simulink model "vfs_matlab"  (R2022a)
settings: Solver=FixedStepAuto  StartTime=0.0  StopTime=tend  FixedStep=0.01  RelTol=1e-3
undefined symbols (not defined in the file): Angle, Axis, center, epsilon, gd, Homogeneous, Kc, pwo_init, scale, SE3, v
libraries: simlib_vpc_basic x23, simlib_vpc_coremath x13, simlib_vpc_gp x3
settings Model: Creator=marco  LastModifiedBy=marco
settings DebuggingCC: AlgebraicLoopMsg=none  ArtificialAlgebraicLoopMsg=none  UnconnectedInputMsg=warning  UnconnectedOutputMsg=warning  UnconnectedLineMsg=warning
settings RTWCC: DLArmComputeVersion=19.05

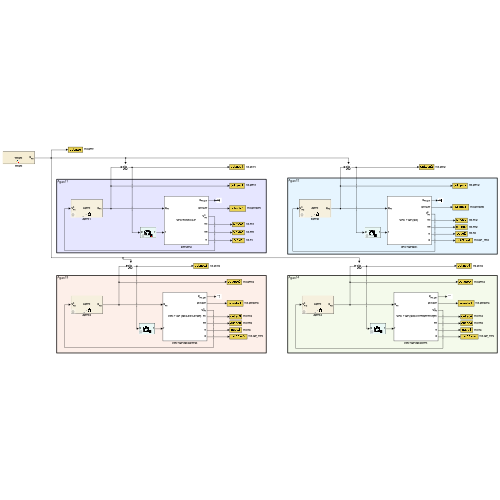
[thumbnail: Simulink's stored preview of the top-level diagram]
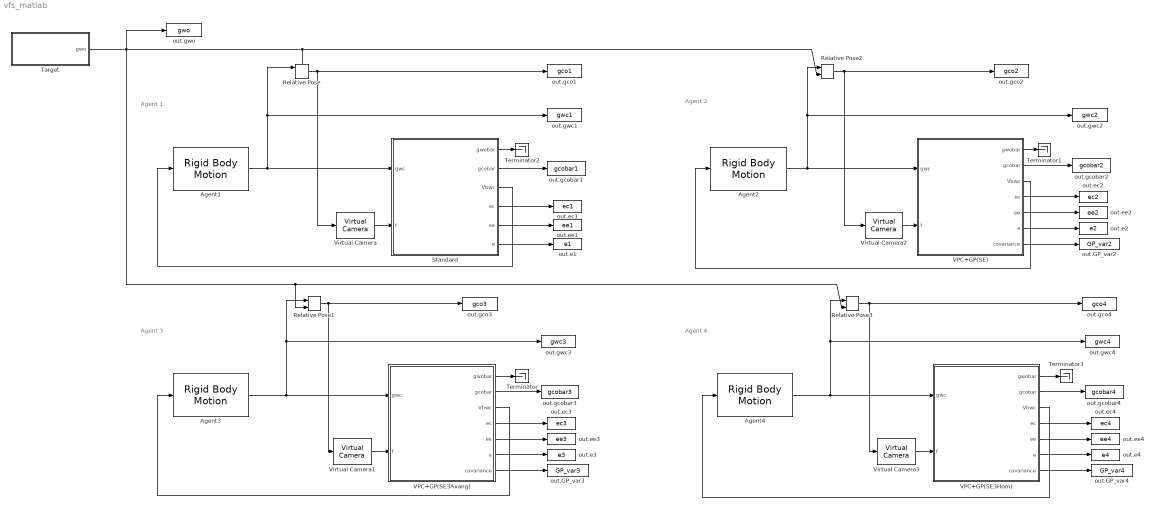
== system vfs_matlab ==
  note: Agent 3
  note: Agent 2
  note: Agent 1
  note: Agent 4
  Agent1 : simlib_vpc_basic/Rigid Body Motion  rbmtype=agent  agentnumber=1  projection=on  show_dg=off  g0=gwc_init
      settings: SourceProductName=VPC Library
  Agent2 : simlib_vpc_basic/Rigid Body Motion  rbmtype=agent  agentnumber=2  projection=on  show_dg=off  g0=gwc_init
      settings: SourceProductName=VPC Library
  Agent3 : simlib_vpc_basic/Rigid Body Motion  rbmtype=agent  agentnumber=3  projection=on  show_dg=off  g0=gwc_init
      settings: SourceProductName=VPC Library
  Agent4 : simlib_vpc_basic/Rigid Body Motion  rbmtype=agent  agentnumber=3  projection=on  show_dg=off  g0=gwc_init
      settings: SourceProductName=VPC Library
  Relative Pose{,1..3} (4 alike) : simlib_vpc_coremath/Relative Pose
      settings: SourceProductName=VPC Library
  Standard : Subsystem
      mask Display:
      | disp('VPC without GP','texmode','on')
      | 
      | % Label ports
      | port_label('input',1,'g_{wc}','texmode','on')
      | port_label('input',2,'f','texmode','on')
      | port_label('output',1,'g_{wo,bar}','texmode','on')
      | port_label('output',2,'gco,bar','texmode','on')
      | port_label('output',3,'V^b_{wc}','texmode','on')
      | port_label('output',4,'ec','texmode','on')
      | port_label('output',5,'ee','texmode','on')
      | port_label('output',6,'e','texmode','on')
  Target : Subsystem
      mask Display:
      | % Glitch in Matlab: If you define a line whose starting point and end point
      | % is equal, then the entire mask block is plotted in bold
      | plot([0,0],[0,0])
      | 
      | % Draw Box
      | plot([0,1,1,0,0],[0,0,1,1,0])
      | 
      | % Write label
      | disp('Target','texmode','on')
      | 
      | % Image
      | p=get_param(gcb,'Position');
      | size = min(p(3:4)-p(1:2));
      | blkscale = abs((p(3)-p(1)) / (p(4)-p(2)));
      | if abs((p(3)-p(1))) > abs((p(4)-p(2))) % block is horizontal
      |     scale = .5*[1/blkscale .6];
      | else % block is vertical
      |     scale = .5*[1 .6*blkscale];
      | end
      | pos = [1-scale(1) 0.1]/2;
      | image('ico_target.png',[pos scale],'off')
      | 
      | % Label ports
      | port_label('output',1,['g_{wo}'],'texmode','on')
  Terminator{,1..3} (4 alike) : Terminator
  VPC+GP(SE) : Subsystem
      mask Display:
      | disp('VPC + GP (SE)','texmode','on')
      | 
      | % Label ports
      | port_label('input',1,'g_{wc}','texmode','on')
      | port_label('input',2,'f','texmode','on')
      | port_label('output',1,'g_{wo,bar}','texmode','on')
      | port_label('output',2,'gco,bar','texmode','on')
      | port_label('output',3,'V^b_{wc}','texmode','on')
      | port_label('output',4,'ec','texmode','on')
      | port_label('output',5,'ee','texmode','on')
      | port_label('output',6,'e','texmode','on')
      | port_label('output',7,'\Sigma','texmode','on')
  VPC+GP(SE3Axang) : Subsystem
      mask Display:
      | disp('VPC + GP (SE3 Axis-Angle)','texmode','on')
      | 
      | % Label ports
      | port_label('input',1,'g_{wc}','texmode','on')
      | port_label('input',2,'f','texmode','on')
      | port_label('output',1,'g_{wo,bar}','texmode','on')
      | port_label('output',2,'gco,bar','texmode','on')
      | port_label('output',3,'V^b_{wc}','texmode','on')
      | port_label('output',4,'ec','texmode','on')
      | port_label('output',5,'ee','texmode','on')
      | port_label('output',6,'e','texmode','on')
      | port_label('output',7,'\Sigma','texmode','on')
  VPC+GP(SE3Hom) : Subsystem
      mask Display:
      | disp('VPC + GP (SE3 Homogeneous)','texmode','on')
      | 
      | % Label ports
      | port_label('input',1,'g_{wc}','texmode','on')
      | port_label('input',2,'f','texmode','on')
      | port_label('output',1,'g_{wo,bar}','texmode','on')
      | port_label('output',2,'gco,bar','texmode','on')
      | port_label('output',3,'V^b_{wc}','texmode','on')
      | port_label('output',4,'ec','texmode','on')
      | port_label('output',5,'ee','texmode','on')
      | port_label('output',6,'e','texmode','on')
      | port_label('output',7,'\Sigma','texmode','on')
  Virtual Camera{,1..3} (4 alike) : simlib_vpc_basic/Virtual Camera  camtype=Pinhole  po=fp  lambda=lambda
      settings: SourceProductName=VPC Library
  out.GP_var2 : ToWorkspace  VariableName=GP_var2  SaveFormat=Structure With Time  SampleTime=-1
  out.GP_var3 : ToWorkspace  VariableName=GP_var3  SaveFormat=Structure With Time  SampleTime=-1
  out.GP_var4 : ToWorkspace  VariableName=GP_var4  SaveFormat=Structure With Time  SampleTime=-1
  out.e1 : ToWorkspace  VariableName=e1  SaveFormat=Structure With Time  SampleTime=-1
  out.e2 : ToWorkspace  VariableName=e2  SaveFormat=Structure With Time  SampleTime=-1
  out.e3 : ToWorkspace  VariableName=e3  SaveFormat=Structure With Time  SampleTime=-1
  out.e4 : ToWorkspace  VariableName=e4  SaveFormat=Structure With Time  SampleTime=-1
  out.ec1 : ToWorkspace  VariableName=ec1  SaveFormat=Structure With Time  SampleTime=-1
  out.ec2 : ToWorkspace  VariableName=ec2  SaveFormat=Structure With Time  SampleTime=-1
  out.ec3 : ToWorkspace  VariableName=ec3  SaveFormat=Structure With Time  SampleTime=-1
  out.ec4 : ToWorkspace  VariableName=ec4  SaveFormat=Structure With Time  SampleTime=-1
  out.ee1 : ToWorkspace  VariableName=ee1  SaveFormat=Structure With Time  SampleTime=-1
  out.ee2 : ToWorkspace  VariableName=ee2  SaveFormat=Structure With Time  SampleTime=-1
  out.ee3 : ToWorkspace  VariableName=ee3  SaveFormat=Structure With Time  SampleTime=-1
  out.ee4 : ToWorkspace  VariableName=ee4  SaveFormat=Structure With Time  SampleTime=-1
  out.gco1 : ToWorkspace  VariableName=gco1  SaveFormat=Structure With Time  SampleTime=-1
  out.gco2 : ToWorkspace  VariableName=gco2  SaveFormat=Structure With Time  SampleTime=-1
  out.gco3 : ToWorkspace  VariableName=gco3  SaveFormat=Structure With Time  SampleTime=-1
  out.gco4 : ToWorkspace  VariableName=gco4  SaveFormat=Structure With Time  SampleTime=-1
  out.gcobar1 : ToWorkspace  VariableName=gcobar1  SaveFormat=Structure With Time  SampleTime=-1
  out.gcobar2 : ToWorkspace  VariableName=gcobar2  SaveFormat=Structure With Time  SampleTime=-1
  out.gcobar3 : ToWorkspace  VariableName=gcobar3  SaveFormat=Structure With Time  SampleTime=-1
  out.gcobar4 : ToWorkspace  VariableName=gcobar4  SaveFormat=Structure With Time  SampleTime=-1
  out.gwc1 : ToWorkspace  VariableName=gwc1  SaveFormat=Structure With Time  SampleTime=-1
  out.gwc2 : ToWorkspace  VariableName=gwc2  SaveFormat=Structure With Time  SampleTime=-1
  out.gwc3 : ToWorkspace  VariableName=gwc3  SaveFormat=Structure With Time  SampleTime=-1
  out.gwc4 : ToWorkspace  VariableName=gwc4  SaveFormat=Structure With Time  SampleTime=-1
  out.gwo : ToWorkspace  VariableName=gwo  SaveFormat=Structure With Time  SampleTime=-1
  wires:
  Relative Pose2/1 -> Virtual Camera2/1, out.gco2/1
  Relative Pose/1 -> Virtual Camera/1, out.gco1/1
  VPC+GP(SE)/2(gcobar) -> out.gcobar2/1
  VPC+GP(SE3Axang)/4(ec) -> out.ec3/1
  Relative Pose1/1 -> out.gco3/1, Virtual Camera1/1
  Agent3/1 -> VPC+GP(SE3Axang)/1(gwc), out.gwc3/1, Relative Pose1/1
  Virtual Camera/1 -> Standard/2(f)
  VPC+GP(SE3Axang)/2(gcobar) -> out.gcobar3/1
  Virtual Camera2/1 -> VPC+GP(SE)/2(f)
  VPC+GP(SE3Axang)/5(ee) -> out.ee3/1
  VPC+GP(SE)/4(ec) -> out.ec2/1
  VPC+GP(SE3Axang)/6(e) -> out.e3/1
  Virtual Camera1/1 -> VPC+GP(SE3Axang)/2(f)
  Agent1/1 -> Standard/1(gwc), out.gwc1/1, Relative Pose/1
  Standard/6(e) -> out.e1/1
  Target/1(gwo) -> out.gwo/1, Relative Pose2/2, Relative Pose/2, Relative Pose3/2, Relative Pose1/2
  Standard/4(ec) -> out.ec1/1
  Standard/5(ee) -> out.ee1/1
  Agent2/1 -> VPC+GP(SE)/1(gwc), out.gwc2/1, Relative Pose2/1
  Standard/2(gcobar) -> out.gcobar1/1
  VPC+GP(SE)/5(ee) -> out.ee2/1
  VPC+GP(SE)/6(e) -> out.e2/1
  Standard/3(Vbwc) -> Agent1/1
  VPC+GP(SE3Axang)/3(Vbwc) -> Agent3/1
  VPC+GP(SE)/3(Vbwc) -> Agent2/1
  VPC+GP(SE3Axang)/1(gwobar) -> Terminator/1
  VPC+GP(SE)/1(gwobar) -> Terminator1/1
  Standard/1(gwobar) -> Terminator2/1
  VPC+GP(SE)/7(covariance) -> out.GP_var2/1
  VPC+GP(SE3Axang)/7(covariance) -> out.GP_var3/1
  VPC+GP(SE3Hom)/6(e) -> out.e4/1
  VPC+GP(SE3Hom)/5(ee) -> out.ee4/1
  VPC+GP(SE3Hom)/2(gcobar) -> out.gcobar4/1
  VPC+GP(SE3Hom)/3(Vbwc) -> Agent4/1
  Virtual Camera3/1 -> VPC+GP(SE3Hom)/2(f)
  Agent4/1 -> VPC+GP(SE3Hom)/1(gwc), Relative Pose3/1, out.gwc4/1
  VPC+GP(SE3Hom)/4(ec) -> out.ec4/1
  Relative Pose3/1 -> Virtual Camera3/1, out.gco4/1
  VPC+GP(SE3Hom)/7(covariance) -> out.GP_var4/1
  VPC+GP(SE3Hom)/1(gwobar) -> Terminator3/1

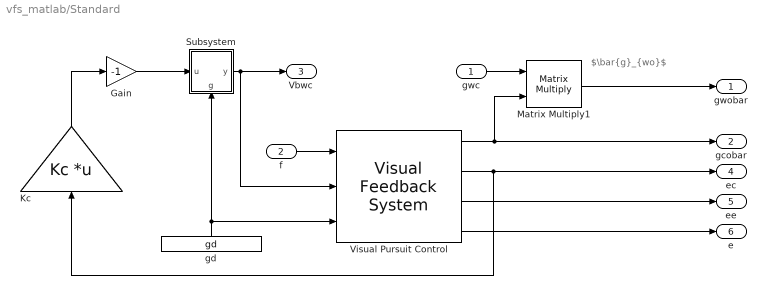
== system vfs_matlab/Standard ==
  note: $\bar{g}_{wo}$
  gwc : Inport
  f : Inport  Port=2
  Gain : Gain  Gain=-1
  Kc : Gain  Gain=Kc  Multiplication=Matrix(K*u) (u vector)
  Matrix Multiply1 : Product  Multiplication=Matrix(*)
  Subsystem : Subsystem
      settings: PortSchema="{\"entries\":[{\"content\":{\"sides\":[{\"content\":{\"connectorIds\":[\"In1\"]},\"type\":\"ConnectorPlacement.EquallySpacedRectSide\",\"uuid\":\"72e68008-5c4a-43a9-a560-64c6a31a0c08\"},{\"content\":{\"connectorIds\":[\"Out1\"],\"side\":\"RIGHT\"},\"type\":\"ConnectorPlacement.EquallySpacedRectSide\",\"uuid\":\"da07f5ff-2b2c-4c55-a2f2-34e133777503\"},{\"content\":{\"connectorIds\":[],\"side\":\"TOP\"},\"type\":\"ConnectorPlacement.EquallySpacedRectSide\",\"uuid\":\"6d174428-4364-4e89-aba7-4e9864808ab5\"},{\"content\":{\"connectorIds\":[\"In2\"],\"side\":\"BOTTOM\"},\"type\":\"ConnectorPlacement.EquallySpacedRectSide\",\"uuid\":\"f9633104-9c11-4d21-90a7-e0f886d9e92d\"},{\"content\":{\"connectorIds\":[],\"side\":\"HIDDEN\"},\"type\":\"ConnectorPlacement.EquallySpacedRectSide\",\"uuid\":\"662f08ae-9279-4a4f-85ea-81d97ead27d9\"}]},\"type\":\"ConnectorPlacement.EquallySpacedConnector\",\"uuid\":\"f3cd156c-cccd-47c6-b81c-6113f78efd58\"}],\"packageUris\":[\"http://schema.mathworks.com/mf0/Connector/R2020b\"],\"version\":\"1.0\"}"
      mask Display:
      | % Glitch in Matlab: If you define a line whose starting point and end point
      | % is equal, then the entire mask block is plotted in bold
      | plot([0,0],[0,0])
      | 
      | % Draw box
      | indent = 0.3;
      | ang=[0:0.2:pi/2, pi/2];
      | plot([0,1-indent],[0,0])
      | xp=indent*sin(ang)+1-indent;
      | yp=indent-indent*cos(ang);
      | plot(xp,yp);
      | plot([1,1,indent],[indent,1,1])
      | xp=indent-indent*sin(ang);
      | yp=1-indent+indent*cos(ang);
      | plot(xp,yp);
      | plot([0,0],[1-indent,0])
      | 
      | % Write label & ports
      | disp('-Ad_{(g_d)}','texmode','on')
      | text(0.5,0.2,'\fontsize{7}g_d','texmode','on')
  Visual Pursuit Control : simlib_vpc_basic/Visual Feedback System  gd_source=external  gd_value=[eye(4,3),ones(4,1)]  gcobar0=gco_init  Ke_source=internal  Ke=Ke  projection=on  camtype=Pinhole  fo=fp  lambda=lambda  show_Vbwo=off  show_ec=on  show_gce=off  show_ee=on  show_gee=off  show_e=on  show_nu=off  show_dgcobar=off  show_ue_aux=off
      settings: SourceProductName=VPC Library
  gd : Constant  Value=gd
  gwobar : Outport
  gcobar : Outport  Port=2
  Vbwc : Outport  Port=3
  ec : Outport  Port=4
  ee : Outport  Port=5
  e : Outport  Port=6
  wires:
  f/1 -> Visual Pursuit Control/1
  Matrix Multiply1/1 -> gwobar/1
  Subsystem/1(y) -> Vbwc/1, Visual Pursuit Control/2
  gwc/1 -> Matrix Multiply1/1
  Kc/1 -> Gain/1
  Visual Pursuit Control/4 -> e/1
  Gain/1 -> Subsystem/1(u)
  Visual Pursuit Control/2 -> ec/1, Kc/1
  Visual Pursuit Control/3 -> ee/1
  gd/1 -> Subsystem/2(g), Visual Pursuit Control/3
  Visual Pursuit Control/1 -> gcobar/1, Matrix Multiply1/2

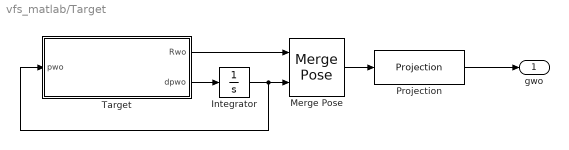
== system vfs_matlab/Target ==
  Integrator : Integrator  InitialCondition=pwo_init  ContinuousStateAttributes='pose'
  Merge Pose : simlib_vpc_coremath/Merge Pose
      settings: SourceProductName=VPC Library
  Projection : simlib_vpc_basic/Projection  projectiontype=averaging  inputtype=pose
      settings: SourceProductName=VPC Library
  Target : MATLAB Function  TreatAsAtomicUnit=on
  gwo : Outport
  wires:
  Merge Pose/1 -> Projection/1
  Projection/1 -> gwo/1
  Integrator/1 -> Target/1(pwo), Merge Pose/2
  Target/2(dpwo) -> Integrator/1
  Target/1(Rwo) -> Merge Pose/1

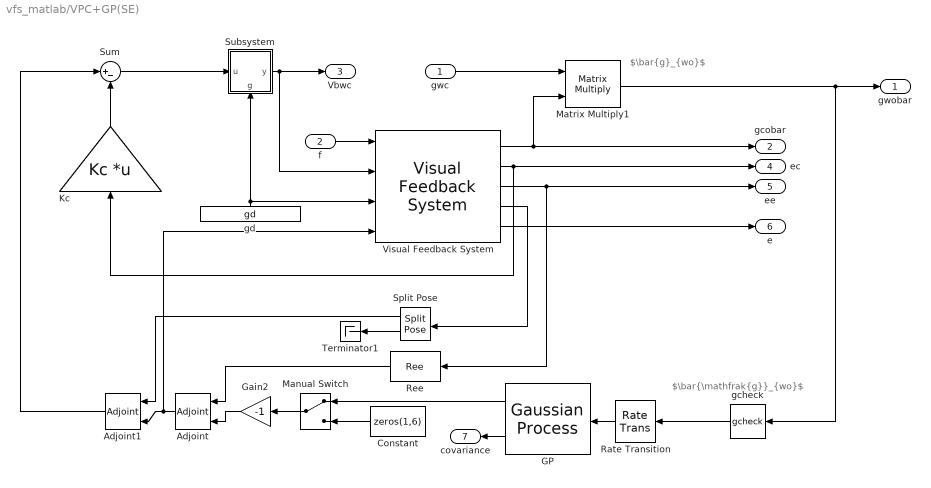
== system vfs_matlab/VPC+GP(SE) ==
  note: $\bar{g}_{wo}$
  note: $\bar{\mathfrak{g}}_{wo}$
  gwc : Inport
  f : Inport  Port=2
  Adjoint : simlib_vpc_basic/Adjoint  adjointtype=orientation
      settings: SourceProductName=VPC Library
  Adjoint1 : simlib_vpc_basic/Adjoint  adjointtype=orientation
      settings: SourceProductName=VPC Library
  Constant : Constant  Value=zeros(1,6)
  GP : simlib_vpc_gp/Gaussian Process  X=X_GP_se  Y=Y_GP_se  sn=sn_GP_se  kernel=Squared Exponential  hyp=hyp_GP_se  show_mean=on  show_variance=on  inv_fallback=off
      settings: SourceProductName=VPC Library
  Gain2 : Gain  Gain=-1
  Kc : Gain  Gain=Kc  Multiplication=Matrix(K*u) (u vector)
  Manual Switch : ManualSwitch
  Matrix Multiply1 : Product  Multiplication=Matrix(*)
  Rate Transition : RateTransition
  Ree : simlib_vpc_coremath/Ree
      settings: SourceProductName=VPC Library
  Split Pose : simlib_vpc_coremath/Split Pose  show_R=on  show_p=on
      settings: SourceProductName=VPC Library
  Subsystem : Subsystem
      settings: PortSchema="{\"entries\":[{\"content\":{\"sides\":[{\"content\":{\"connectorIds\":[\"In1\"]},\"type\":\"ConnectorPlacement.EquallySpacedRectSide\",\"uuid\":\"72e68008-5c4a-43a9-a560-64c6a31a0c08\"},{\"content\":{\"connectorIds\":[\"Out1\"],\"side\":\"RIGHT\"},\"type\":\"ConnectorPlacement.EquallySpacedRectSide\",\"uuid\":\"da07f5ff-2b2c-4c55-a2f2-34e133777503\"},{\"content\":{\"connectorIds\":[],\"side\":\"TOP\"},\"type\":\"ConnectorPlacement.EquallySpacedRectSide\",\"uuid\":\"6d174428-4364-4e89-aba7-4e9864808ab5\"},{\"content\":{\"connectorIds\":[\"In2\"],\"side\":\"BOTTOM\"},\"type\":\"ConnectorPlacement.EquallySpacedRectSide\",\"uuid\":\"f9633104-9c11-4d21-90a7-e0f886d9e92d\"},{\"content\":{\"connectorIds\":[],\"side\":\"HIDDEN\"},\"type\":\"ConnectorPlacement.EquallySpacedRectSide\",\"uuid\":\"662f08ae-9279-4a4f-85ea-81d97ead27d9\"}]},\"type\":\"ConnectorPlacement.EquallySpacedConnector\",\"uuid\":\"f3cd156c-cccd-47c6-b81c-6113f78efd58\"}],\"packageUris\":[\"http://schema.mathworks.com/mf0/Connector/R2020b\"],\"version\":\"1.0\"}"
      mask Display:
      | % Glitch in Matlab: If you define a line whose starting point and end point
      | % is equal, then the entire mask block is plotted in bold
      | plot([0,0],[0,0])
      | 
      | % Draw box
      | indent = 0.3;
      | ang=[0:0.2:pi/2, pi/2];
      | plot([0,1-indent],[0,0])
      | xp=indent*sin(ang)+1-indent;
      | yp=indent-indent*cos(ang);
      | plot(xp,yp);
      | plot([1,1,indent],[indent,1,1])
      | xp=indent-indent*sin(ang);
      | yp=1-indent+indent*cos(ang);
      | plot(xp,yp);
      | plot([0,0],[1-indent,0])
      | 
      | % Write label & ports
      | disp('-Ad_{(g_d)}','texmode','on')
      | text(0.5,0.2,'\fontsize{7}g_d','texmode','on')
  Sum : Sum  Inputs=|+-
  Terminator1 : Terminator
  Visual Feedback System : simlib_vpc_basic/Visual Feedback System  gd_source=external  gd_value=[eye(4,3),ones(4,1)]  gcobar0=gco_init  Ke_source=internal  Ke=Ke  projection=on  camtype=Pinhole  fo=fp  lambda=lambda  show_Vbwo=off  show_ec=on  show_gce=on  show_ee=on  show_gee=off  show_e=on  show_nu=off  show_dgcobar=off  show_ue_aux=on
      settings: SourceProductName=VPC Library
  gcheck : simlib_vpc_coremath/gcheck
      settings: SourceProductName=VPC Library
  gd : Constant  Value=gd
  gwobar : Outport
  gcobar : Outport  Port=2
  Vbwc : Outport  Port=3
  ec : Outport  Port=4
  ee : Outport  Port=5
  e : Outport  Port=6
  covariance : Outport  Port=7
  wires:
  f/1 -> Visual Feedback System/1
  Matrix Multiply1/1 -> gcheck/1, gwobar/1
  Subsystem/1(y) -> Vbwc/1, Visual Feedback System/2
  gwc/1 -> Matrix Multiply1/1
  Visual Feedback System/5 -> e/1
  Kc/1 -> Sum/2
  Visual Feedback System/2 -> ec/1, Kc/1
  Visual Feedback System/3 -> Ree/1, ee/1
  gd/1 -> Subsystem/2(g), Visual Feedback System/3
  Visual Feedback System/1 -> Matrix Multiply1/2, gcobar/1
  Split Pose/1 -> Adjoint1/2
  Rate Transition/1 -> GP/1
  Adjoint/1 -> Visual Feedback System/4, Adjoint1/1
  Ree/1 -> Adjoint/2
  Split Pose/2 -> Terminator1/1
  Gain2/1 -> Adjoint/1
  Manual Switch/1 -> Gain2/1
  Sum/1 -> Subsystem/1(u)
  Adjoint1/1 -> Sum/1
  Visual Feedback System/4 -> Split Pose/1
  gcheck/1 -> Rate Transition/1
  GP/1 -> Manual Switch/1
  Constant/1 -> Manual Switch/2
  GP/2 -> covariance/1

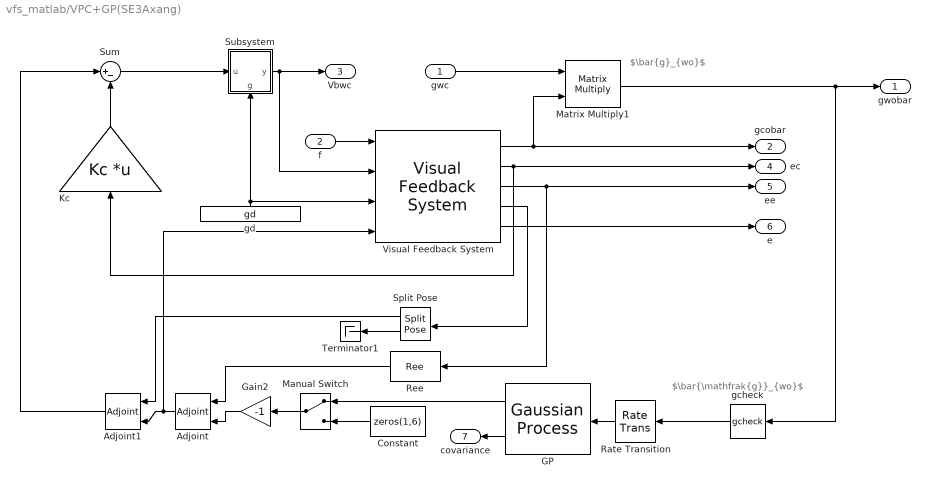
== system vfs_matlab/VPC+GP(SE3Axang) ==
  note: $\bar{g}_{wo}$
  note: $\bar{\mathfrak{g}}_{wo}$
  gwc : Inport
  f : Inport  Port=2
  Adjoint : simlib_vpc_basic/Adjoint  adjointtype=orientation
      settings: SourceProductName=VPC Library
  Adjoint1 : simlib_vpc_basic/Adjoint  adjointtype=orientation
      settings: SourceProductName=VPC Library
  Constant : Constant  Value=zeros(1,6)
  GP : simlib_vpc_gp/Gaussian Process  X=X_GP_axang  Y=Y_GP_axang  sn=sn_GP_axang  kernel=SE3 (Axis-Angle)  hyp=hyp_GP_axang  show_mean=on  show_variance=on  inv_fallback=on
      settings: SourceProductName=VPC Library
  Gain2 : Gain  Gain=-1
  Kc : Gain  Gain=Kc  Multiplication=Matrix(K*u) (u vector)
  Manual Switch : ManualSwitch
  Matrix Multiply1 : Product  Multiplication=Matrix(*)
  Rate Transition : RateTransition
  Ree : simlib_vpc_coremath/Ree
      settings: SourceProductName=VPC Library
  Split Pose : simlib_vpc_coremath/Split Pose  show_R=on  show_p=on
      settings: SourceProductName=VPC Library
  Subsystem : Subsystem
      settings: PortSchema="{\"entries\":[{\"content\":{\"sides\":[{\"content\":{\"connectorIds\":[\"In1\"]},\"type\":\"ConnectorPlacement.EquallySpacedRectSide\",\"uuid\":\"72e68008-5c4a-43a9-a560-64c6a31a0c08\"},{\"content\":{\"connectorIds\":[\"Out1\"],\"side\":\"RIGHT\"},\"type\":\"ConnectorPlacement.EquallySpacedRectSide\",\"uuid\":\"da07f5ff-2b2c-4c55-a2f2-34e133777503\"},{\"content\":{\"connectorIds\":[],\"side\":\"TOP\"},\"type\":\"ConnectorPlacement.EquallySpacedRectSide\",\"uuid\":\"6d174428-4364-4e89-aba7-4e9864808ab5\"},{\"content\":{\"connectorIds\":[\"In2\"],\"side\":\"BOTTOM\"},\"type\":\"ConnectorPlacement.EquallySpacedRectSide\",\"uuid\":\"f9633104-9c11-4d21-90a7-e0f886d9e92d\"},{\"content\":{\"connectorIds\":[],\"side\":\"HIDDEN\"},\"type\":\"ConnectorPlacement.EquallySpacedRectSide\",\"uuid\":\"662f08ae-9279-4a4f-85ea-81d97ead27d9\"}]},\"type\":\"ConnectorPlacement.EquallySpacedConnector\",\"uuid\":\"f3cd156c-cccd-47c6-b81c-6113f78efd58\"}],\"packageUris\":[\"http://schema.mathworks.com/mf0/Connector/R2020b\"],\"version\":\"1.0\"}"
      mask Display:
      | % Glitch in Matlab: If you define a line whose starting point and end point
      | % is equal, then the entire mask block is plotted in bold
      | plot([0,0],[0,0])
      | 
      | % Draw box
      | indent = 0.3;
      | ang=[0:0.2:pi/2, pi/2];
      | plot([0,1-indent],[0,0])
      | xp=indent*sin(ang)+1-indent;
      | yp=indent-indent*cos(ang);
      | plot(xp,yp);
      | plot([1,1,indent],[indent,1,1])
      | xp=indent-indent*sin(ang);
      | yp=1-indent+indent*cos(ang);
      | plot(xp,yp);
      | plot([0,0],[1-indent,0])
      | 
      | % Write label & ports
      | disp('-Ad_{(g_d)}','texmode','on')
      | text(0.5,0.2,'\fontsize{7}g_d','texmode','on')
  Sum : Sum  Inputs=|+-
  Terminator1 : Terminator
  Visual Feedback System : simlib_vpc_basic/Visual Feedback System  gd_source=external  gd_value=[eye(4,3),ones(4,1)]  gcobar0=gco_init  Ke_source=internal  Ke=Ke  projection=on  camtype=Pinhole  fo=fp  lambda=lambda  show_Vbwo=off  show_ec=on  show_gce=on  show_ee=on  show_gee=off  show_e=on  show_nu=off  show_dgcobar=off  show_ue_aux=on
      settings: SourceProductName=VPC Library
  gcheck : simlib_vpc_coremath/gcheck
      settings: SourceProductName=VPC Library
  gd : Constant  Value=gd
  gwobar : Outport
  gcobar : Outport  Port=2
  Vbwc : Outport  Port=3
  ec : Outport  Port=4
  ee : Outport  Port=5
  e : Outport  Port=6
  covariance : Outport  Port=7
  wires:
  f/1 -> Visual Feedback System/1
  Matrix Multiply1/1 -> gcheck/1, gwobar/1
  Subsystem/1(y) -> Vbwc/1, Visual Feedback System/2
  gwc/1 -> Matrix Multiply1/1
  Visual Feedback System/5 -> e/1
  Kc/1 -> Sum/2
  Visual Feedback System/2 -> ec/1, Kc/1
  Visual Feedback System/3 -> Ree/1, ee/1
  gd/1 -> Subsystem/2(g), Visual Feedback System/3
  Visual Feedback System/1 -> Matrix Multiply1/2, gcobar/1
  Split Pose/1 -> Adjoint1/2
  Rate Transition/1 -> GP/1
  Adjoint/1 -> Visual Feedback System/4, Adjoint1/1
  Ree/1 -> Adjoint/2
  Split Pose/2 -> Terminator1/1
  Gain2/1 -> Adjoint/1
  Manual Switch/1 -> Gain2/1
  Sum/1 -> Subsystem/1(u)
  Adjoint1/1 -> Sum/1
  Visual Feedback System/4 -> Split Pose/1
  gcheck/1 -> Rate Transition/1
  GP/1 -> Manual Switch/1
  Constant/1 -> Manual Switch/2
  GP/2 -> covariance/1

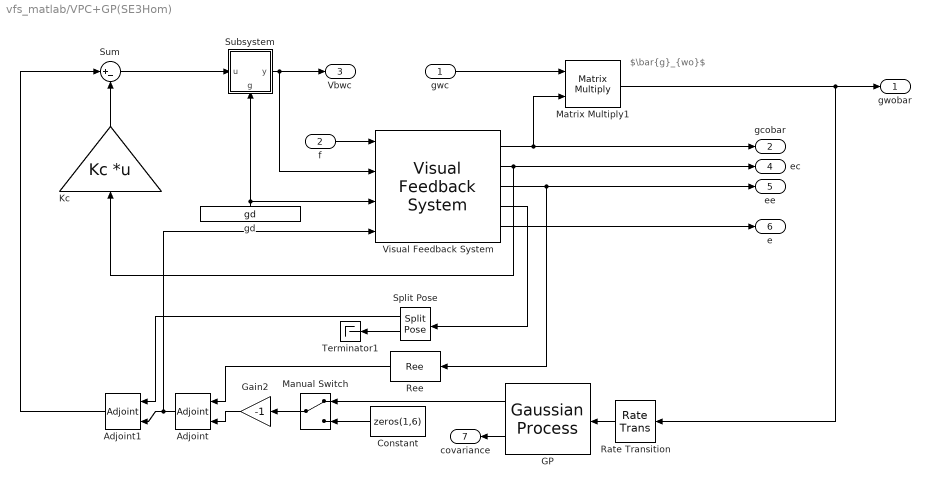
== system vfs_matlab/VPC+GP(SE3Hom) ==
  note: $\bar{g}_{wo}$
  gwc : Inport
  f : Inport  Port=2
  Adjoint : simlib_vpc_basic/Adjoint  adjointtype=orientation
      settings: SourceProductName=VPC Library
  Adjoint1 : simlib_vpc_basic/Adjoint  adjointtype=orientation
      settings: SourceProductName=VPC Library
  Constant : Constant  Value=zeros(1,6)
  GP : simlib_vpc_gp/Gaussian Process  X=X_GP_hom  Y=Y_GP_hom  sn=sn_GP_hom  kernel=SE3 (Homogeneous)  hyp=hyp_GP_hom  show_mean=on  show_variance=on  inv_fallback=off
      settings: SourceProductName=VPC Library
  Gain2 : Gain  Gain=-1
  Kc : Gain  Gain=Kc  Multiplication=Matrix(K*u) (u vector)
  Manual Switch : ManualSwitch
  Matrix Multiply1 : Product  Multiplication=Matrix(*)
  Rate Transition : RateTransition
  Ree : simlib_vpc_coremath/Ree
      settings: SourceProductName=VPC Library
  Split Pose : simlib_vpc_coremath/Split Pose  show_R=on  show_p=on
      settings: SourceProductName=VPC Library
  Subsystem : Subsystem
      settings: PortSchema="{\"entries\":[{\"content\":{\"sides\":[{\"content\":{\"connectorIds\":[\"In1\"]},\"type\":\"ConnectorPlacement.EquallySpacedRectSide\",\"uuid\":\"72e68008-5c4a-43a9-a560-64c6a31a0c08\"},{\"content\":{\"connectorIds\":[\"Out1\"],\"side\":\"RIGHT\"},\"type\":\"ConnectorPlacement.EquallySpacedRectSide\",\"uuid\":\"da07f5ff-2b2c-4c55-a2f2-34e133777503\"},{\"content\":{\"connectorIds\":[],\"side\":\"TOP\"},\"type\":\"ConnectorPlacement.EquallySpacedRectSide\",\"uuid\":\"6d174428-4364-4e89-aba7-4e9864808ab5\"},{\"content\":{\"connectorIds\":[\"In2\"],\"side\":\"BOTTOM\"},\"type\":\"ConnectorPlacement.EquallySpacedRectSide\",\"uuid\":\"f9633104-9c11-4d21-90a7-e0f886d9e92d\"},{\"content\":{\"connectorIds\":[],\"side\":\"HIDDEN\"},\"type\":\"ConnectorPlacement.EquallySpacedRectSide\",\"uuid\":\"662f08ae-9279-4a4f-85ea-81d97ead27d9\"}]},\"type\":\"ConnectorPlacement.EquallySpacedConnector\",\"uuid\":\"f3cd156c-cccd-47c6-b81c-6113f78efd58\"}],\"packageUris\":[\"http://schema.mathworks.com/mf0/Connector/R2020b\"],\"version\":\"1.0\"}"
      mask Display:
      | % Glitch in Matlab: If you define a line whose starting point and end point
      | % is equal, then the entire mask block is plotted in bold
      | plot([0,0],[0,0])
      | 
      | % Draw box
      | indent = 0.3;
      | ang=[0:0.2:pi/2, pi/2];
      | plot([0,1-indent],[0,0])
      | xp=indent*sin(ang)+1-indent;
      | yp=indent-indent*cos(ang);
      | plot(xp,yp);
      | plot([1,1,indent],[indent,1,1])
      | xp=indent-indent*sin(ang);
      | yp=1-indent+indent*cos(ang);
      | plot(xp,yp);
      | plot([0,0],[1-indent,0])
      | 
      | % Write label & ports
      | disp('-Ad_{(g_d)}','texmode','on')
      | text(0.5,0.2,'\fontsize{7}g_d','texmode','on')
  Sum : Sum  Inputs=|+-
  Terminator1 : Terminator
  Visual Feedback System : simlib_vpc_basic/Visual Feedback System  gd_source=external  gd_value=[eye(4,3),ones(4,1)]  gcobar0=gco_init  Ke_source=internal  Ke=Ke  projection=on  camtype=Pinhole  fo=fp  lambda=lambda  show_Vbwo=off  show_ec=on  show_gce=on  show_ee=on  show_gee=off  show_e=on  show_nu=off  show_dgcobar=off  show_ue_aux=on
      settings: SourceProductName=VPC Library
  gd : Constant  Value=gd
  gwobar : Outport
  gcobar : Outport  Port=2
  Vbwc : Outport  Port=3
  ec : Outport  Port=4
  ee : Outport  Port=5
  e : Outport  Port=6
  covariance : Outport  Port=7
  wires:
  Constant/1 -> Manual Switch/2
  GP/1 -> Manual Switch/1
  Matrix Multiply1/1 -> Rate Transition/1, gwobar/1
  Visual Feedback System/4 -> Split Pose/1
  Adjoint1/1 -> Sum/1
  Sum/1 -> Subsystem/1(u)
  Manual Switch/1 -> Gain2/1
  Gain2/1 -> Adjoint/1
  Split Pose/2 -> Terminator1/1
  Ree/1 -> Adjoint/2
  Adjoint/1 -> Adjoint1/1, Visual Feedback System/4
  Rate Transition/1 -> GP/1
  Split Pose/1 -> Adjoint1/2
  Visual Feedback System/1 -> gcobar/1, Matrix Multiply1/2
  gd/1 -> Visual Feedback System/3, Subsystem/2(g)
  Visual Feedback System/3 -> ee/1, Ree/1
  Visual Feedback System/2 -> Kc/1, ec/1
  Kc/1 -> Sum/2
  Visual Feedback System/5 -> e/1
  gwc/1 -> Matrix Multiply1/1
  Subsystem/1(y) -> Visual Feedback System/2, Vbwc/1
  f/1 -> Visual Feedback System/1
  GP/2 -> covariance/1

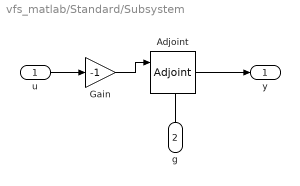
== system vfs_matlab/Standard/Subsystem ==
  u : Inport
  g : Inport  Port=2
  Adjoint : simlib_vpc_basic/Adjoint  adjointtype=pose
      settings: SourceProductName=VPC Library
  Gain : Gain  Gain=-1
  y : Outport
  wires:
  Adjoint/1 -> y/1
  u/1 -> Gain/1
  g/1 -> Adjoint/2
  Gain/1 -> Adjoint/1

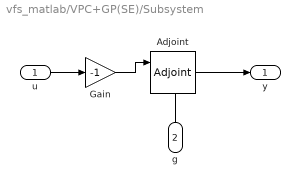
== system vfs_matlab/VPC+GP(SE)/Subsystem ==
  u : Inport
  g : Inport  Port=2
  Adjoint : simlib_vpc_basic/Adjoint  adjointtype=pose
      settings: SourceProductName=VPC Library
  Gain : Gain  Gain=-1
  y : Outport
  wires:
  Adjoint/1 -> y/1
  u/1 -> Gain/1
  g/1 -> Adjoint/2
  Gain/1 -> Adjoint/1

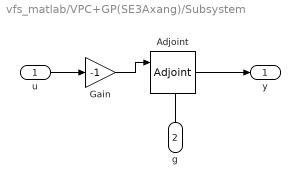
== system vfs_matlab/VPC+GP(SE3Axang)/Subsystem ==
  u : Inport
  g : Inport  Port=2
  Adjoint : simlib_vpc_basic/Adjoint  adjointtype=pose
      settings: SourceProductName=VPC Library
  Gain : Gain  Gain=-1
  y : Outport
  wires:
  Adjoint/1 -> y/1
  u/1 -> Gain/1
  g/1 -> Adjoint/2
  Gain/1 -> Adjoint/1

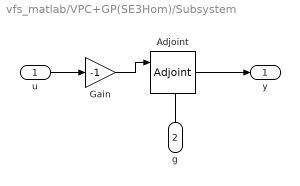
== system vfs_matlab/VPC+GP(SE3Hom)/Subsystem ==
  u : Inport
  g : Inport  Port=2
  Adjoint : simlib_vpc_basic/Adjoint  adjointtype=pose
      settings: SourceProductName=VPC Library
  Gain : Gain  Gain=-1
  y : Outport
  wires:
  Gain/1 -> Adjoint/1
  g/1 -> Adjoint/2
  u/1 -> Gain/1
  Adjoint/1 -> y/1

== matlab function vfs_matlab/Target/Target ==
  data: pwo input; v parameter; Rwo output; dpwo output; epsilon parameter; scale parameter; center parameter
function [Rwo, dpwo] = target_trajectory(pwo, v, epsilon, scale, center) %#codegen
% Target Movement
%
% Editor:
%   OMAINSKA Marco - Doctoral Student, Cybernetics
%       <marcoomainska@g.ecc.u-tokyo.ac.jp>
% Review:
%   YAMAUCHI Junya - Assistant Professor
%       <junya_yamauchi@ipc.i.u-tokyo.ac.jp>
%
% Property of: Fujita-Yamauchi Lab, University of Tokyo, 2023
% Website: https://www.scl.ipc.i.u-tokyo.ac.jp
%
%------------- BEGIN CODE --------------

% Get velocity
% Vb = vanderpol(pwo,v,epsilon,center,scale);
Vb = quartic(pwo,v,epsilon,center,scale);
dpwo = Vb(1:3);

% set heading angle
zangle = rad2deg(atan2(dpwo(2),dpwo(1)) - pi/2);
alpha = rad2deg(asin( dpwo(3)/norm(dpwo,2) ));
Rwo = rotz(zangle)*rotx(alpha);

%------------- END CODE --------------
end
